simulink model "DUST4_Nonlinear_Airframe"  (R2024b)
settings: Solver=VariableStepAuto  StartTime=0.0  StopTime=10.0  RelTol=1e-3
undefined symbols (not defined in the file or in its folder): AC, Aero, mot, prop, rad, s, Vbi
libraries: aerolibasang x3, aerolibconvert2 x3, aerolibactuator x3, shared6dof x2, aerolibtransform2 x2, aerolibadyn x1, vrlib x1
(part 2 of 2)

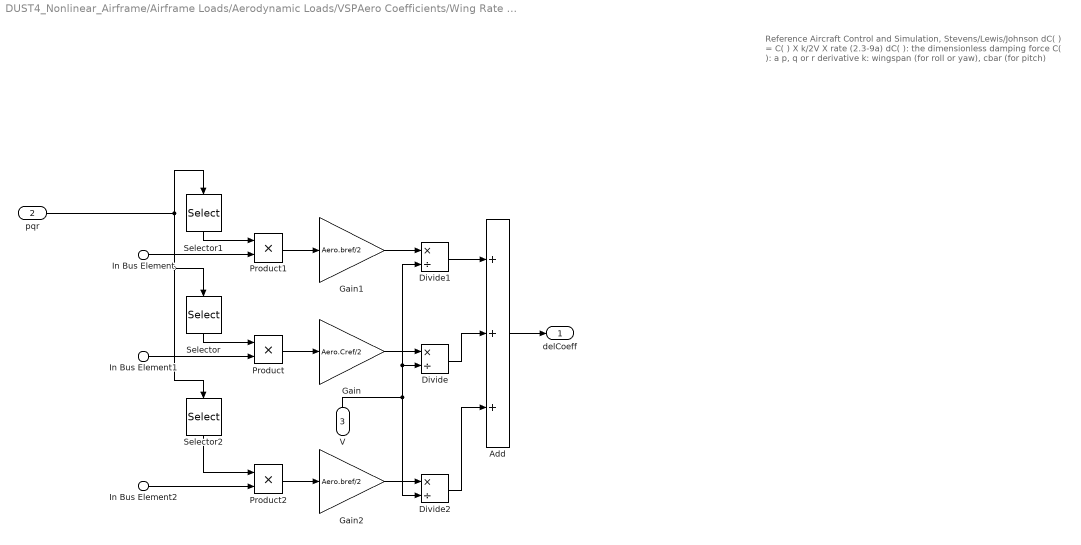
== system DUST4_Nonlinear_Airframe/Airframe Loads/Aerodynamic Loads/VSPAero Coefficients/Wing Rate Effects/Aero Surfaces/Convert & Add ==
  note: Reference Aircraft Control and Simulation, Stevens/Lewis/Johnson
      | dC( ) = C( ) X k/2V X rate    (2.3-9a)
      |
      | dC( ): the dimensionless damping force
      | C( ): a p, q or r derivative
      | k: wingspan (for roll or yaw), cbar (for pitch)
  In Bus Element : Inport  PortName=DampCoef  Element=C()_p
  In Bus Element1 : Inport  PortName=DampCoef  Element=C()_q
  In Bus Element2 : Inport  PortName=DampCoef  Element=C()_r
  pqr : Inport  Port=2
  V : Inport  Port=3
  Add : Sum  Inputs=+++
  Divide : Product  Inputs=*/
  Divide1 : Product  Inputs=*/
  Divide2 : Product  Inputs=*/
  Gain : Gain  Gain=Aero.Cref/2
  Gain1 : Gain  Gain=Aero.bref/2
  Gain2 : Gain  Gain=Aero.bref/2
  Product : Product
  Product1 : Product
  Product2 : Product
  Selector : Selector  InputPortWidth=3  IndexOptions=Index vector (dialog)  Indices=[ 2]  OutputSizes=1
  Selector1 : Selector  InputPortWidth=3  IndexOptions=Index vector (dialog)  Indices=[ 1]  OutputSizes=1
  Selector2 : Selector  InputPortWidth=3  IndexOptions=Index vector (dialog)  Indices=[ 3]  OutputSizes=1
  delCoeff : Outport
  wires:
  pqr/1 -> Selector1/1, Selector2/1, Selector/1
  Divide1/1 -> Add/1
  Selector/1 -> Product/1
  Selector1/1 -> Product1/1
  Gain1/1 -> Divide1/1
  Product1/1 -> Gain1/1
  Gain/1 -> Divide/1
  V/1 -> Divide2/2, Divide1/2, Divide/2
  Product/1 -> Gain/1
  In Bus Element2/1 -> Product2/2
  Divide/1 -> Add/2
  Divide2/1 -> Add/3
  Gain2/1 -> Divide2/1
  Product2/1 -> Gain2/1
  Add/1 -> delCoeff/1
  In Bus Element1/1 -> Product/2
  Selector2/1 -> Product2/1
  In Bus Element/1 -> Product1/2
